simulink model "Q5_Simulink"  (Simulink 9.1)
settings: Solver=VariableStepAuto  StartTime=0.0  StopTime=10.0  RelTol=1e-3
settings Model: Creator=acer  LastModifiedBy=acer
settings DataIOCC: SaveFormat=Dataset
settings OptimizationCC: LifeSpan=auto
settings DebuggingCC: UnderspecifiedInitializationDetection=Simplified  MergeDetectMultiDrivingBlocksExec=error  SFUnexpectedBacktrackingDiag=error  SFNoUnconditionalDefaultTransitionDiag=error  SFExecutionAtInitializationDiag=warning
settings HardwareCC: ProdBitPerPointer=64  ProdBitPerSizeT=64  ProdBitPerPtrDiffT=64  ProdLargestAtomicFloat=Float  ProdIntDivRoundTo=Zero  ProdEndianess=LittleEndian  ProdWordSize=64  ProdHWDeviceType=Intel->x86-64 (Windows64)
settings ModelReferenceCC: PropagateSignalLabelsOutOfModel=on
settings CodeAppCC: StateflowObjectComments=off
settings GRTTargetCC: TargetLangStandard=C99 (ISO)  CombineOutputUpdateFcns=on  GRTInterface=off
settings ConfigComp: CovMetricSettings=dwe  CovHtmlReporting=off  CovSaveCumulativeToWorkspaceVar=off  CovSaveSingleToWorkspaceVar=off  CovExternalEMLEnable=on

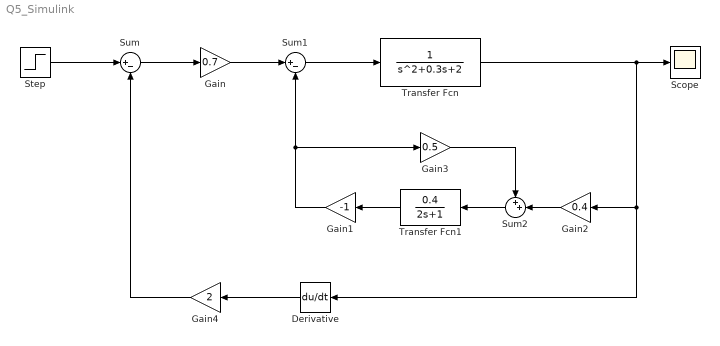
== system Q5_Simulink ==
  Derivative : Derivative
  Gain : Gain  Gain=0.7
  Gain1 : Gain  Gain=-1
  Gain2 : Gain  Gain=0.4
  Gain3 : Gain  Gain=0.5
  Gain4 : Gain  Gain=2
  Scope : Scope
  Step : Step  SampleTime=0
  Sum : Sum  Inputs=|+-
  Sum1 : Sum  Inputs=|+-
  Sum2 : Sum  Inputs=++|
  Transfer Fcn : TransferFcn  Denominator=[1 0.3 2]
  Transfer Fcn1 : TransferFcn  Numerator=[0.4]  Denominator=[2 1]
  wires:
  Transfer Fcn/1 -> Derivative/1, Gain2/1, Scope/1
  Gain4/1 -> Sum/2
  Step/1 -> Sum/1
  Sum/1 -> Gain/1
  Gain/1 -> Sum1/1
  Sum1/1 -> Transfer Fcn/1
  Gain1/1 -> Gain3/1, Sum1/2
  Transfer Fcn1/1 -> Gain1/1
  Gain3/1 -> Sum2/1
  Gain2/1 -> Sum2/2
  Sum2/1 -> Transfer Fcn1/1
  Derivative/1 -> Gain4/1
